simulink model "SSI_Simulink"  (R2020b)
settings: Solver=FixedStepAuto  StartTime=0.0  StopTime=inf  RelTol=1e-3
undefined symbols (not defined in the file): serial
libraries: instrumentlib x3
settings Model: EnablePacing=on  Creator=pavlo  LastModifiedBy=pavlo
settings RTWCC: Description=Simulink Desktop Real-Time  SystemTargetFile=sldrt.tlc  TemplateMakefile=sldrt.tmf  RTWCompilerOptimization=on
settings CodeAppCC: MaxIdLength=95
settings SimulinkDesktopRealTimeCC: TargetPreCompLibLocation=D:\MATLAB R2020b\toolbox\sldrt\lib\win64

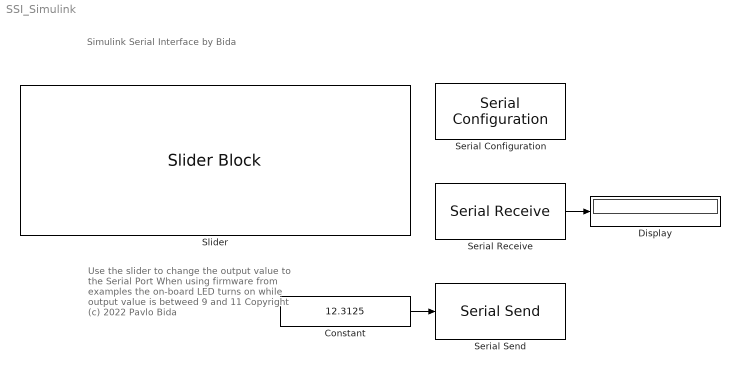
== system SSI_Simulink ==
  note: Simulink Serial Interface by Bida
  note: Use the slider to change the output value to the Serial Port
      |
      | When using firmware from examples
      | the on-board LED turns on while output value is betweed 9 and 11
      |
      | Copyright (c) 2022 Pavlo Bida
  Constant : Constant  Value=12.3125  OutDataTypeStr=single  SampleTime=0.01
  Display : Display
  Serial Configuration : instrumentlib/Serial Configuration  Priority=-200000  ComPortMenu=<Please select a port...>  ComPort=COM4  ObjConstructor=serial('COM4');  BaudRate=115200  DataBits=8  Parity=none  StopBits=1  FlowControl=none  Timeout=10  ByteOrder=LittleEndian
  Serial Receive : instrumentlib/Serial Receive  ComPortMenu=<Please select a port...>  ComPort=COM4  ObjConstructor=serial('COM4');  Terminator=<none>  DataSize=[1 1]  DataType=single  EnableBlockingMode=on  ActionDataUnavailable=Output last received value  CustomValue=0  SampleTime=0.01
  Serial Send : instrumentlib/Serial Send  ComPortMenu=<Please select a port...>  ComPort=COM4  ObjConstructor=serial('COM4');  Terminator=<none>  EnableBlockingMode=off
  Slider : SliderBlock  ScaleMax=20
  wires:
  Serial Receive/1 -> Display/1
  Constant/1 -> Serial Send/1
